simulink model "comparison_px4_mc_sim_distrb_ekf"  (R2019b)
settings: Solver=FixedStepAuto  StartTime=0.0  StopTime=sim_time  FixedStep=1/sim_freq  RelTol=1e-3
values from neighbouring files (symbols this model uses):
  C_D = [0.064; 0.067; 0.089].*0    [full_distrb_model_parameters.m]    (also in model_parameters.m)
  d = 0.11    [full_distrb_model_parameters.m]    (also in model_parameters.m)
  disturbance_rejection = 1    [full_performance_analysis.m]    (also in performance_analysis.m)
  hover_perc = m*g / max_total_T    [full_distrb_model_parameters.m]    (also in model_parameters.m)
  Ixx = 1.326e-3    (= 0.001326)    [full_distrb_model_parameters.m]    (also in model_parameters.m)
  Iyy = 9.3e-4    (= 0.00093)    [full_distrb_model_parameters.m]    (also in model_parameters.m)
  Izz = 1.95e-3    (= 0.00195)    [full_distrb_model_parameters.m]    (also in model_parameters.m)
  m = 0.66    [full_distrb_model_parameters.m]    (also in model_parameters.m)
  max_T = max_total_T / 4    [full_distrb_model_parameters.m]    (also in model_parameters.m)
  meas_noise = 0.000001    (= 1e-06)    [full_distrb_model_parameters.m]    (also in full_performance_analysis.m; model_parameters.m; noise_matrices.m = 0.0001; run_sim_full_dstrb.m)
  option1 = 3    [full_performance_analysis.m]    (also in performance_analysis.m)
  option2 = 2    [full_performance_analysis.m]    (also in performance_analysis.m = 1)
  Pk_init = zeros(15)    [full_distrb_model_parameters.m]    (also in full_performance_analysis.m; model_parameters.m = zeros(12); noise_matrices.m = zeros(12,12); run_sim_full_dstrb.m)
  pos_e_step = [0,0,0]    [full_performance_analysis.m]    (also in performance_analysis.m; run_sim.m = [0,2,0]; run_sim_full_dstrb.m)
  Qk = C22'*C12    [full_distrb_model_parameters.m]    (also in full_performance_analysis.m; model_parameters.m; noise_matrices.m; run_sim_full_dstrb.m)
  r_D = 7.997e-3    (= 0.007997)    [full_distrb_model_parameters.m]    (also in model_parameters.m)
  ramp_max = 0.15    [full_performance_analysis.m]    (also in performance_analysis.m; run_sim.m = 0.5; run_sim_full_dstrb.m = 0.1)
  ramp_slope = 0.05    [full_performance_analysis.m]    (also in performance_analysis.m; run_sim.m; run_sim_full_dstrb.m = 0.01)
  Rk = eye(9)*meas_noise    [full_distrb_model_parameters.m]    (also in full_performance_analysis.m; model_parameters.m; noise_matrices.m; run_sim_full_dstrb.m)
  sinus_amplitude = 0.2    [full_performance_analysis.m]    (also in performance_analysis.m; run_sim.m = 0.1; run_sim_full_dstrb.m = 0.1)
  sinus_bias = 0    [full_performance_analysis.m]    (also in performance_analysis.m; run_sim.m; run_sim_full_dstrb.m)
  sinus_freq = 3    [full_performance_analysis.m]    (also in performance_analysis.m = 5; run_sim.m = 1; run_sim_full_dstrb.m = 10)
  step_delay = 3    [full_performance_analysis.m]    (also in performance_analysis.m; run_sim.m = 1; run_sim_full_dstrb.m = 1)
  step_mag = 0.1    [full_performance_analysis.m]    (also in performance_analysis.m; run_sim.m = 0.5; run_sim_full_dstrb.m)
  tau_T = 0.002    [full_distrb_model_parameters.m]    (also in model_parameters.m)
  virtual_controls_mat = [1 1 1 1; -1/sqrt(2) 1/sqrt(2) 1/sqrt(2) -1/sqrt(2); 1/sqrt(2) -1/sqrt(2) 1/sqrt(2) -1/sqrt(2); 1 1 -1 -1]    [full_distrb_model_parameters.m]    (also in model_parameters.m)
  wind = [0; 0; 0]    [full_distrb_model_parameters.m]    (also in model_parameters.m)
  X_hat_init = zeros(15,1)    [full_distrb_model_parameters.m]    (also in full_performance_analysis.m; model_parameters.m = zeros(12,1); noise_matrices.m = zeros(12,1); run_sim_full_dstrb.m)
  yaw_step = 0    [full_performance_analysis.m]    (also in performance_analysis.m; run_sim.m; run_sim_full_dstrb.m)
undefined symbols (not defined in the file or in its folder): br_filt_denom, br_filt_num, DiscIntNeverNeededParam, eta_w, g, MC_PITCH_P, MC_PITCHRATE_D, MC_PITCHRATE_I, MC_PITCHRATE_MAX, MC_PITCHRATE_P, MC_PR_INT_LIM, MC_ROLL_P, MC_ROLLRATE_D, MC_ROLLRATE_I, MC_ROLLRATE_MAX, MC_ROLLRATE_P, MC_RR_INT_LIM, MC_YAW_P, MC_YAWRATE_D, MC_YAWRATE_I, MC_YAWRATE_MAX, MC_YAWRATE_P, MC_YR_INT_LIM, MPC_THR_MAX, MPC_THR_MIN, MPC_TILTMAX_AIR, MPC_XY_P, MPC_XY_VEL_D, MPC_XY_VEL_I, MPC_XY_VEL_MAX, MPC_XY_VEL_P, MPC_Z_P, MPC_Z_VEL_D, MPC_Z_VEL_I, MPC_Z_VEL_MAX_DN, MPC_Z_VEL_MAX_UP, MPC_Z_VEL_P, rho, sim_freq, vel_filt_denom, vel_filt_num
libraries: simulink x7, sharedtransform x3, shared6dof x1
settings Model: Creator=henry  LastModifiedBy=henry

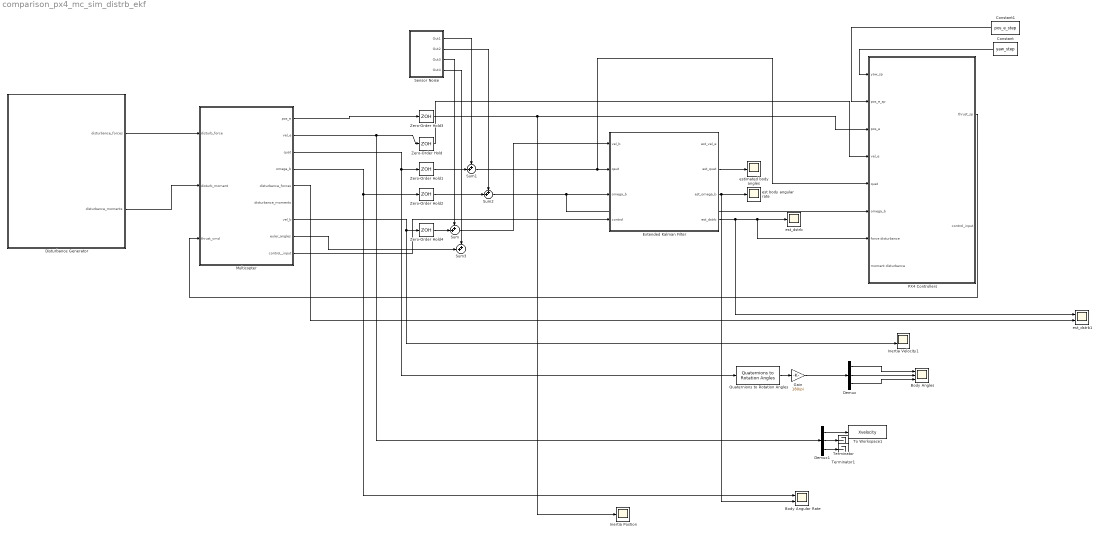
== system comparison_px4_mc_sim_distrb_ekf ==
  Body Angles : Scope  NumInputPorts=3
  Body Angular Rate : Scope  NumInputPorts=2
  Constant : Constant  Value=yaw_step
  Constant1 : Constant  Value=pos_e_step
  Demux : Demux  Outputs=3
  Demux1 : Demux  Outputs=3
  Disturbance Generator : Subsystem
  Extended Kalman Filter : Subsystem
  Gain : Gain  Gain=180/pi
  Inertia Postion : Scope
  Inertia Velocity1 : Scope  NumInputPorts=2
  Multicopter : Subsystem
  PX4 Controllers : Subsystem
  Quaternions to Rotation Angles : sharedtransform/Quaternions to Rotation Angles  rotationOrder=XYZ  aMode=aMode
      settings: SourceProductBaseCode=AE
  "Sensor Noise " : Subsystem
  Sum{,1..3} (4 alike) : Sum  Inputs=++|
  Terminator : Terminator
  Terminator1 : Terminator
  To Workspace1 : ToWorkspace  VariableName=Xvelocity  SaveFormat=Timeseries  SampleTime=-1
  Zero-Order Hold{,1..4} (5 alike) : ZeroOrderHold  SampleTime=1/sim_freq
  est body angular rate : Scope
  est_dstrb : Scope
  est_dstrb1 : Scope  NumInputPorts=2
  estimated body angles : Scope
  wires:
  Multicopter/4(omega_b) -> Body Angular Rate/1, Zero-Order Hold2/1
  Multicopter/1(pos_e) -> Zero-Order Hold3/1
  PX4 Controllers/1(thrust_sp) -> Multicopter/3(thrust_cmd)
  Constant/1 -> PX4 Controllers/1(yaw_sp)
  Constant1/1 -> PX4 Controllers/2(pos_e_sp)
  Quaternions to Rotation Angles/1 -> Gain/1
  Gain/1 -> Demux/1
  Demux/1 -> Body Angles/1
  Demux/2 -> Body Angles/2
  Demux/3 -> Body Angles/3
  Zero-Order Hold2/1 -> Sum2/2
  Sum2/1 -> PX4 Controllers/6(omega_b), Extended Kalman Filter/3(omega_b)
  Zero-Order Hold3/1 -> Inertia Postion/1, PX4 Controllers/3(pos_e)
  Multicopter/3("quat ") -> Quaternions to Rotation Angles/1, Zero-Order Hold1/1
  Multicopter/7("vel_b ") -> Inertia Velocity1/2, Zero-Order Hold4/1
  Zero-Order Hold4/1 -> Sum/2
  Sum/1 -> Extended Kalman Filter/1(vel_b)
  Zero-Order Hold/1 -> PX4 Controllers/4(vel_e)
  Extended Kalman Filter/3(est_omega_b) -> est body angular rate/1, Body Angular Rate/2
  Extended Kalman Filter/2(est_quat) -> estimated body angles/1
  Multicopter/8(euler_angles) -> Sum3/2
  Multicopter/9(controL_input) -> Extended Kalman Filter/4(control)
  Multicopter/2(vel_e) -> Demux1/1, Zero-Order Hold/1
  Zero-Order Hold1/1 -> Sum1/2
  Sum1/1 -> PX4 Controllers/5(quat), Extended Kalman Filter/2(qaut)
  Extended Kalman Filter/4(est_dstrb) -> est_dstrb1/1, PX4 Controllers/7(force disturbance), est_dstrb/1
  Multicopter/5(disturbance_forces) -> est_dstrb1/2
  Disturbance Generator/1(disturbance_forces) -> Multicopter/1(disturb_force)
  Disturbance Generator/2(disturbance_moments) -> Multicopter/2(disturb_moment)
  Demux1/2 -> Terminator/1
  Demux1/3 -> Terminator1/1
  Demux1/1 -> To Workspace1/1
  "Sensor Noise "/1(Out1) -> Sum1/1
  "Sensor Noise "/2(Out2) -> Sum2/1
  "Sensor Noise "/3(Out3) -> Sum/1
  "Sensor Noise "/4(Out4) -> Sum3/1

== system comparison_px4_mc_sim_distrb_ekf/Disturbance Generator ==
  note: RAMP
  note: DISTURBANCE TYPE
  note: STEP
  note: SINUS
  note: ACTIVATE DISTURBANCE
  MATLAB Function : MATLAB Function  TreatAsAtomicUnit=on
  Option1 : Constant  Value=option1  OutDataTypeStr=Inherit: Inherit via back propagation
  Option2 : Constant  Value=option2  OutDataTypeStr=Inherit: Inherit via back propagation
  Product : Product
  Ramp : simulink/Sources/Ramp  slope=ramp_slope  start=step_delay  InitialOutput=0
  Saturation : Saturate  UpperLimit=ramp_max  LowerLimit=0
  Sine Wave1 : Sin  Amplitude=sinus_amplitude  Bias=sinus_bias  Frequency=sinus_freq  SampleTime=0
  Step1 : Step  Time=step_delay  After=step_mag  SampleTime=0
  Step2 : Step  Time=step_delay  SampleTime=0
  activate disturbance : Constant  OutDataTypeStr=Inherit: Inherit via back propagation
  disturbance_forces : Outport
  disturbance_moments : Outport  Port=2
  wires:
  Sine Wave1/1 -> Product/1
  Step1/1 -> MATLAB Function/2(step)
  MATLAB Function/2(moments) -> disturbance_moments/1
  Product/1 -> MATLAB Function/4(sinus)
  activate disturbance/1 -> MATLAB Function/1(x)
  Option1/1 -> MATLAB Function/5(option1)
  Option2/1 -> MATLAB Function/6(option2)
  Ramp/1 -> Saturation/1
  MATLAB Function/1(forces) -> disturbance_forces/1
  Saturation/1 -> MATLAB Function/3(ramp)
  Step2/1 -> Product/2

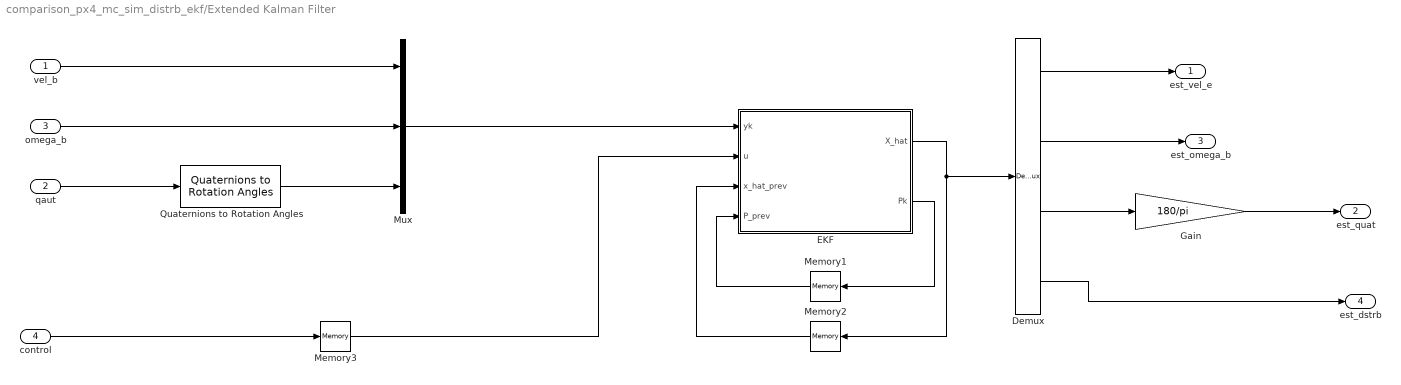
== system comparison_px4_mc_sim_distrb_ekf/Extended Kalman Filter ==
  vel_b : Inport
  qaut : Inport  Port=2
  omega_b : Inport  Port=3
  control : Inport  Port=4
  Demux : Demux
  EKF : MATLAB Function  TreatAsAtomicUnit=on
  Gain : Gain  Gain=180/pi
  Memory1 : Memory  InitialCondition=Pk_init
  Memory2 : Memory  InitialCondition=X_hat_init
  Memory3 : Memory  InitialCondition=[0 0 0 0]'
  Mux : Mux  Inputs=3
  Quaternions to Rotation Angles : sharedtransform/Quaternions to Rotation Angles  rotationOrder=XYZ  aMode=aMode
      settings: SourceProductBaseCode=AE
  est_vel_e : Outport
  est_quat : Outport  Port=2
  est_omega_b : Outport  Port=3
  est_dstrb : Outport  Port=4
  wires:
  qaut/1 -> Quaternions to Rotation Angles/1
  vel_b/1 -> Mux/1
  omega_b/1 -> Mux/2
  Mux/1 -> EKF/1(yk)
  control/1 -> Memory3/1
  Memory1/1 -> EKF/4(P_prev)
  EKF/2(Pk) -> Memory1/1
  EKF/1(X_hat) -> Memory2/1, Demux/1
  Memory2/1 -> EKF/3(x_hat_prev)
  Demux/1 -> est_vel_e/1
  Demux/2 -> est_omega_b/1
  Memory3/1 -> EKF/2(u)
  Quaternions to Rotation Angles/1 -> Mux/3
  Demux/3 -> Gain/1
  Gain/1 -> est_quat/1
  Demux/4 -> est_dstrb/1

== system comparison_px4_mc_sim_distrb_ekf/Multicopter ==
  disturb_force : Inport
  disturb_moment : Inport  Port=2
  thrust_cmd : Inport  Port=3
  6 DOF MODEL : Subsystem
  Forces and Moments : Subsystem
  Motor Model : Subsystem
  pos_e : Outport
  vel_e : Outport  Port=2
  "quat " : Outport  Port=3
  omega_b : Outport  Port=4
  disturbance_forces : Outport  Port=5
  disturbance_moments : Outport  Port=6
  "vel_b " : Outport  Port=7
  euler_angles : Outport  Port=8
  controL_input : Outport  Port=9
  wires:
  6 DOF MODEL/1(vel_b) -> "vel_b "/1, Forces and Moments/1(vel_b)
  6 DOF MODEL/3(qaut) -> Forces and Moments/3(quat), "quat "/1
  6 DOF MODEL/2(pos_e) -> pos_e/1, Forces and Moments/2(pos_e)
  Forces and Moments/2(moments) -> 6 DOF MODEL/2(moments)
  6 DOF MODEL/5(omega_b) -> omega_b/1
  6 DOF MODEL/4(vel_e) -> vel_e/1
  Forces and Moments/1(forces) -> 6 DOF MODEL/1("forces ")
  thrust_cmd/1 -> Motor Model/1(thrust_cmd)
  Motor Model/1(force) -> Forces and Moments/4(thrust_cmd)
  Forces and Moments/3(disturbance_force) -> disturbance_forces/1
  Forces and Moments/4(disturbance_moments) -> disturbance_moments/1
  disturb_force/1 -> Forces and Moments/5(disturb_force)
  disturb_moment/1 -> Forces and Moments/6(disturb_moments)
  6 DOF MODEL/6(euler_angles) -> euler_angles/1
  Forces and Moments/5(control_input) -> controL_input/1

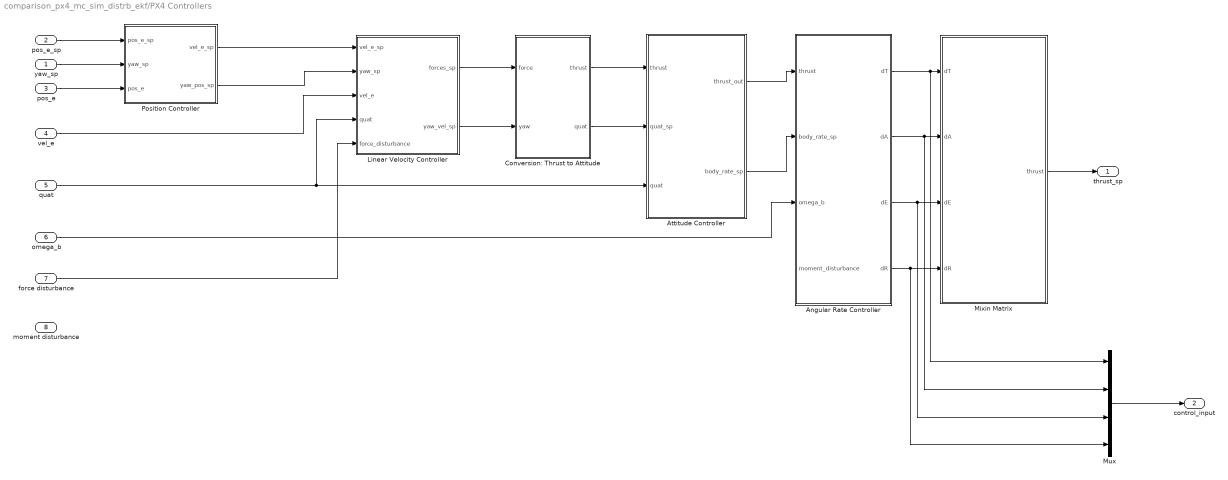
== system comparison_px4_mc_sim_distrb_ekf/PX4 Controllers ==
  yaw_sp : Inport
  pos_e_sp : Inport  Port=2
  pos_e : Inport  Port=3
  vel_e : Inport  Port=4
  quat : Inport  Port=5
  omega_b : Inport  Port=6
  force disturbance : Inport  Port=7
  moment disturbance : Inport  Port=8
  Angular Rate Controller : Subsystem
  Attitude Controller : Subsystem
  Conversion: Thrust to Attitude : Subsystem
  Linear Velocity Controller : Subsystem
  Mixin Matrix : Subsystem
  Mux : Mux
  Position Controller : Subsystem
  thrust_sp : Outport
  control_input : Outport  Port=2  PortDimensions=[4 1]
  wires:
  yaw_sp/1 -> Position Controller/2(yaw_sp)
  pos_e_sp/1 -> Position Controller/1(pos_e_sp)
  quat/1 -> Attitude Controller/3(quat), Linear Velocity Controller/4("quat ")
  omega_b/1 -> Angular Rate Controller/3(omega_b)
  pos_e/1 -> Position Controller/3(pos_e)
  vel_e/1 -> Linear Velocity Controller/3(vel_e)
  Position Controller/2(yaw_pos_sp) -> Linear Velocity Controller/2(yaw_sp)
  Position Controller/1(vel_e_sp) -> Linear Velocity Controller/1(vel_e_sp)
  Linear Velocity Controller/1(forces_sp) -> Conversion: Thrust to Attitude/1(force)
  Linear Velocity Controller/2(yaw_vel_sp) -> Conversion: Thrust to Attitude/2(yaw)
  Conversion: Thrust to Attitude/1(thrust) -> Attitude Controller/1(thrust)
  Conversion: Thrust to Attitude/2(quat) -> Attitude Controller/2(quat_sp)
  Attitude Controller/1(thrust_out) -> Angular Rate Controller/1(thrust)
  Attitude Controller/2(body_rate_sp) -> Angular Rate Controller/2(body_rate_sp)
  Angular Rate Controller/1(dT) -> Mux/1, Mixin Matrix/1(dT)
  Angular Rate Controller/2(dA) -> Mux/2, Mixin Matrix/2(dA)
  Angular Rate Controller/3(dE) -> Mux/3, Mixin Matrix/3(dE)
  Angular Rate Controller/4(dR) -> Mux/4, Mixin Matrix/4(dR)
  Mixin Matrix/1(thrust) -> thrust_sp/1
  Mux/1 -> control_input/1
  force disturbance/1 -> Linear Velocity Controller/5(force_disturbance)

== system comparison_px4_mc_sim_distrb_ekf/Sensor Noise  ==
  Random Number : RandomNumber  Mean=[ 0 0 0 ]  Variance=[meas_noise meas_noise meas_noise]  Seed=[4 5 6 ]  SampleTime=1/sim_freq  VectorParams1D=off
  Random Number1 : RandomNumber  Mean=[0 0 0]  Variance=[meas_noise meas_noise meas_noise]  Seed=[1 2 3]  SampleTime=1/sim_freq  VectorParams1D=off
  Random Number2 : RandomNumber  Mean=[0 0 0]  Variance=[meas_noise meas_noise meas_noise]  Seed=[8 9 10]  SampleTime=1/sim_freq
  Random Number3 : RandomNumber  Mean=[0 0 0 0]  Variance=[meas_noise meas_noise meas_noise meas_noise]  Seed=[11 12 13 14]  SampleTime=1/sim_freq
  Out1 : Outport
  Out2 : Outport  Port=2
  Out3 : Outport  Port=3
  Out4 : Outport  Port=4
  wires:
  Random Number3/1 -> Out1/1
  Random Number/1 -> Out4/1
  Random Number2/1 -> Out3/1
  Random Number1/1 -> Out2/1

== system comparison_px4_mc_sim_distrb_ekf/Multicopter/6 DOF MODEL ==
  "forces " : Inport
  moments : Inport  Port=2
  6DOF (Quaternion) : shared6dof/6DOF (Euler Angles)  units=Metric (MKS)  mtype=Fixed  rep=Quaternion  xme_0=[0 0 0]  Vm_0=[0 0 0]  eul_0=[0 0 0]  pm_0=[0 0 0]  mass_0=m  mass_e=0.5  mass_f=2.0  inertia=I  inertia_e=eye(3)  inertia_f=2*eye(3)  k_quat=2  vre_flag=on  abi_flag=off  aMode=0  xme_statename=''  Vm_statename=''  eul_statename=''  quat_statename=''  pm_statename=''  mass_statename=''
      settings: SourceProductBaseCode=AE
  Direction Cosine Matrix to Quaternions : sharedtransform/Direction Cosine Matrix  to Quaternions  aMode=0  action=None  tolerance=eps(2)
      settings: SourceProductName=Aerospace Blockset  SourceProductBaseCode=AE
  Terminator : Terminator
  Terminator1 : Terminator
  vel_b : Outport
  pos_e : Outport  Port=2
  qaut : Outport  Port=3
  vel_e : Outport  Port=4
  omega_b : Outport  Port=5
  euler_angles : Outport  Port=6
  wires:
  "forces "/1 -> 6DOF (Quaternion)/1
  moments/1 -> 6DOF (Quaternion)/2
  6DOF (Quaternion)/8 -> Terminator/1
  6DOF (Quaternion)/7 -> Terminator1/1
  6DOF (Quaternion)/3 -> euler_angles/1
  6DOF (Quaternion)/1 -> vel_e/1
  6DOF (Quaternion)/2 -> pos_e/1
  6DOF (Quaternion)/5 -> vel_b/1
  6DOF (Quaternion)/6 -> omega_b/1
  Direction Cosine Matrix to Quaternions/1 -> qaut/1
  6DOF (Quaternion)/4 -> Direction Cosine Matrix to Quaternions/1

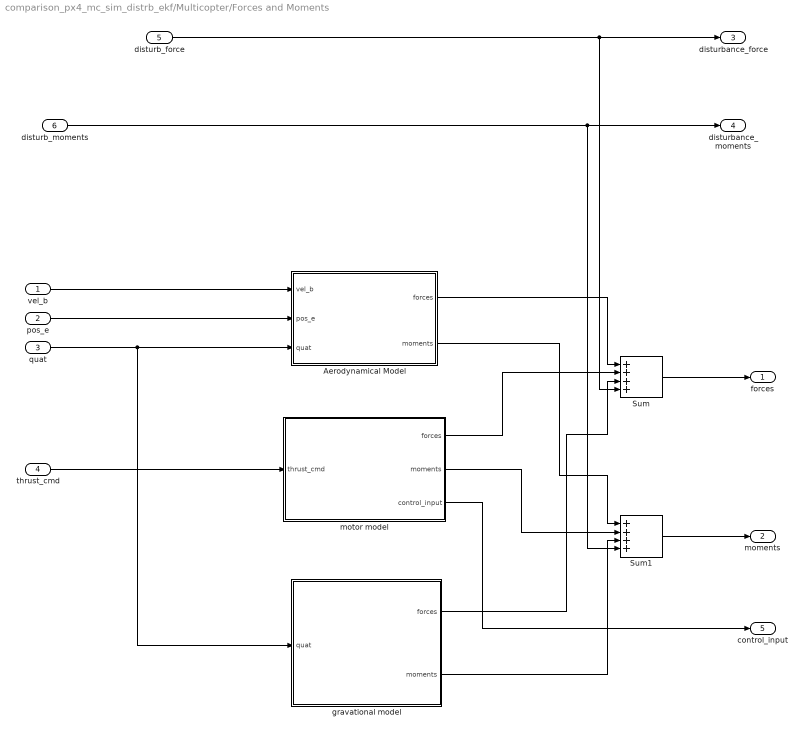
== system comparison_px4_mc_sim_distrb_ekf/Multicopter/Forces and Moments ==
  vel_b : Inport
  pos_e : Inport  Port=2
  quat : Inport  Port=3
  thrust_cmd : Inport  Port=4
  disturb_force : Inport  Port=5
  disturb_moments : Inport  Port=6
  Aerodynamical Model : Subsystem
  Sum : Sum  Inputs=++++
  Sum1 : Sum  Inputs=++++
  gravational model : Subsystem
  motor model : Subsystem
  forces : Outport
  moments : Outport  Port=2
  disturbance_force : Outport  Port=3
  disturbance_moments : Outport  Port=4
  control_input : Outport  Port=5
  wires:
  Sum/1 -> forces/1
  Sum1/1 -> moments/1
  motor model/1(forces) -> Sum/2
  motor model/2(moments) -> Sum1/2
  gravational model/1(forces) -> Sum/3
  gravational model/2(moments) -> Sum1/3
  vel_b/1 -> Aerodynamical Model/1(vel_b)
  pos_e/1 -> Aerodynamical Model/2(pos_e)
  Aerodynamical Model/1(forces) -> Sum/1
  Aerodynamical Model/2(moments) -> Sum1/1
  thrust_cmd/1 -> motor model/1(thrust_cmd)
  disturb_moments/1 -> Sum1/4, disturbance_moments/1
  quat/1 -> Aerodynamical Model/3(quat), gravational model/1(quat)
  disturb_force/1 -> Sum/4, disturbance_force/1
  motor model/3(control_input) -> control_input/1

== system comparison_px4_mc_sim_distrb_ekf/Multicopter/Motor Model ==
  thrust_cmd : Inport
  Linear Gain : Gain  Gain=max_T
  force : Outport  VectorParamsAs1DForOutWhenUnconnected=off
  wires:
  thrust_cmd/1 -> Linear Gain/1
  Linear Gain/1 -> force/1

== system comparison_px4_mc_sim_distrb_ekf/PX4 Controllers/Angular Rate Controller ==
  thrust : Inport
  body_rate_sp : Inport  Port=2
  omega_b : Inport  Port=3
  moment_disturbance : Inport  Port=4
  Demux : Demux  Outputs=3
  Demux1 : Demux  Outputs=3
  Demux2 : Demux  Outputs=3
  Pitch Rate Controller : Subsystem
  Roll Rate Controller : Subsystem
  Yaw Rate Controller : Subsystem
  dT : Outport  VectorParamsAs1DForOutWhenUnconnected=off
  dA : Outport  Port=2  VectorParamsAs1DForOutWhenUnconnected=off
  dE : Outport  Port=3  VectorParamsAs1DForOutWhenUnconnected=off
  dR : Outport  Port=4  VectorParamsAs1DForOutWhenUnconnected=off
  wires:
  Demux1/3 -> Yaw Rate Controller/2(r)
  Demux/3 -> Yaw Rate Controller/1(rref)
  Demux1/1 -> Roll Rate Controller/2(p)
  thrust/1 -> dT/1
  Yaw Rate Controller/1(dR) -> dR/1
  Pitch Rate Controller/1(dE) -> dE/1
  Demux1/2 -> Pitch Rate Controller/2(q)
  Roll Rate Controller/1(dA) -> dA/1
  Demux/1 -> Roll Rate Controller/1(pref)
  Demux/2 -> Pitch Rate Controller/1(qref)
  omega_b/1 -> Demux1/1
  body_rate_sp/1 -> Demux/1
  moment_disturbance/1 -> Demux2/1
  Demux2/2 -> Pitch Rate Controller/3(disturbance_q)
  Demux2/3 -> Yaw Rate Controller/3(disturbance_r)
  Demux2/1 -> Roll Rate Controller/3(disturbance_q)

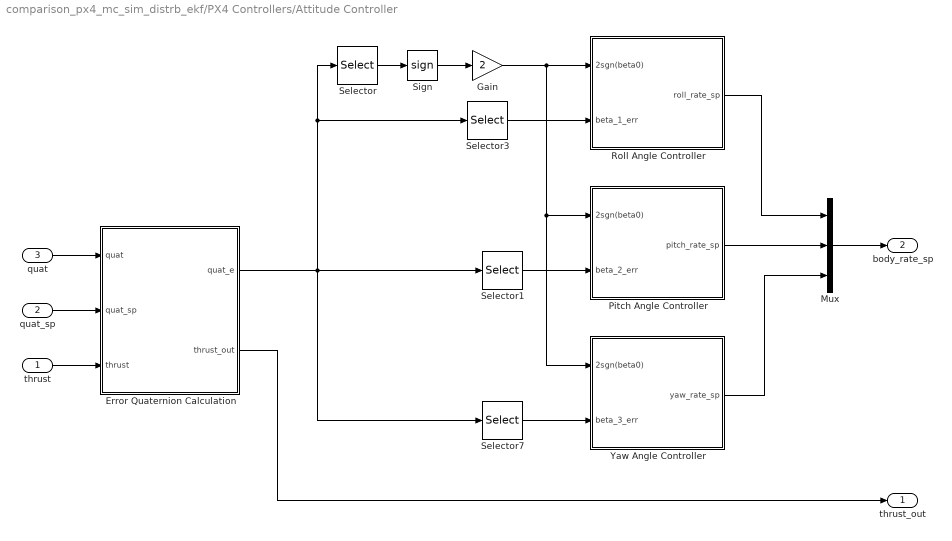
== system comparison_px4_mc_sim_distrb_ekf/PX4 Controllers/Attitude Controller ==
  thrust : Inport  PortDimensions=1
  quat_sp : Inport  Port=2  PortDimensions=4
  quat : Inport  Port=3  PortDimensions=4
  Error Quaternion Calculation : MATLAB Function  TreatAsAtomicUnit=on
  Gain : Gain  Gain=2
  Mux : Mux  Inputs=3
  Pitch Angle Controller : Subsystem
  Roll Angle Controller : Subsystem
  Selector : Selector  InputPortWidth=4  IndexOptions=Index vector (dialog)  Indices=1  OutputSizes=1
  Selector1 : Selector  InputPortWidth=4  IndexOptions=Index vector (dialog)  Indices=3  OutputSizes=1
  Selector3 : Selector  InputPortWidth=4  IndexOptions=Index vector (dialog)  Indices=2  OutputSizes=1
  Selector7 : Selector  InputPortWidth=4  IndexOptions=Index vector (dialog)  Indices=4  OutputSizes=1
  Sign : Signum
  Yaw Angle Controller : Subsystem
  thrust_out : Outport  VectorParamsAs1DForOutWhenUnconnected=off
  body_rate_sp : Outport  Port=2  VectorParamsAs1DForOutWhenUnconnected=off
  wires:
  Pitch Angle Controller/1(pitch_rate_sp) -> Mux/2
  Selector7/1 -> Yaw Angle Controller/2(beta_3_err)
  Mux/1 -> body_rate_sp/1
  quat/1 -> Error Quaternion Calculation/1(quat)
  quat_sp/1 -> Error Quaternion Calculation/2(quat_sp)
  Error Quaternion Calculation/1(quat_e) -> Selector7/1, Selector/1, Selector3/1, Selector1/1
  Selector/1 -> Sign/1
  Yaw Angle Controller/1(yaw_rate_sp) -> Mux/3
  Roll Angle Controller/1(roll_rate_sp) -> Mux/1
  Selector3/1 -> Roll Angle Controller/2(beta_1_err)
  Gain/1 -> Yaw Angle Controller/1(2sgn(beta0)), Pitch Angle Controller/1(2sgn(beta0)), Roll Angle Controller/1(2sgn(beta0))
  thrust/1 -> Error Quaternion Calculation/3(thrust)
  Sign/1 -> Gain/1
  Error Quaternion Calculation/2(thrust_out) -> thrust_out/1
  Selector1/1 -> Pitch Angle Controller/2(beta_2_err)

== system comparison_px4_mc_sim_distrb_ekf/PX4 Controllers/Conversion: Thrust to Attitude ==
  force : Inport
  yaw : Inport  Port=2
  thrust2att : MATLAB Function  TreatAsAtomicUnit=on
  thrust : Outport  VectorParamsAs1DForOutWhenUnconnected=off
  quat : Outport  Port=2  VectorParamsAs1DForOutWhenUnconnected=off
  wires:
  yaw/1 -> thrust2att/2(yaw)
  force/1 -> thrust2att/1(force)
  thrust2att/2(thrust) -> thrust/1
  thrust2att/1(quat) -> quat/1

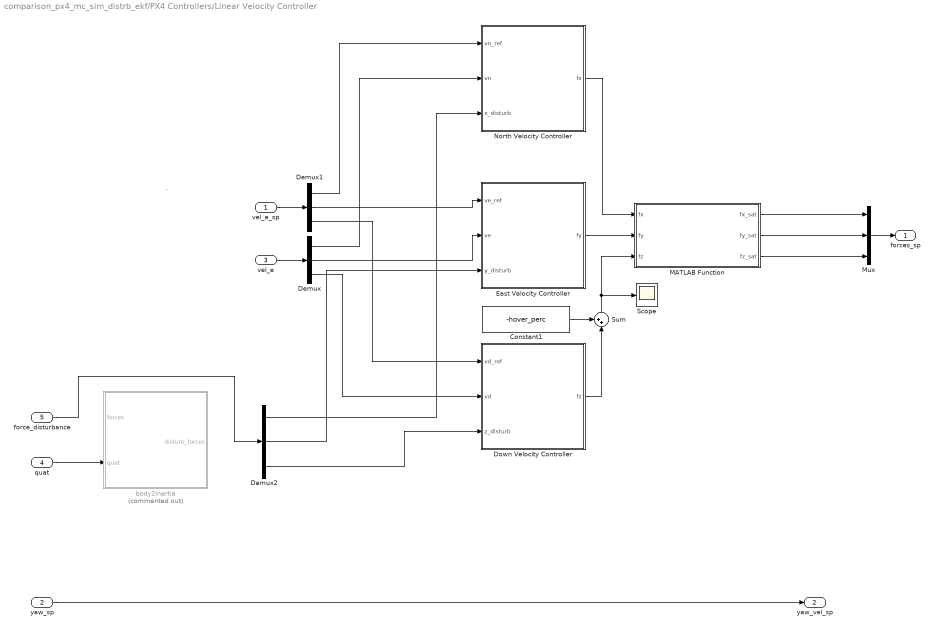
== system comparison_px4_mc_sim_distrb_ekf/PX4 Controllers/Linear Velocity Controller ==
  note: `
  vel_e_sp : Inport
  yaw_sp : Inport  Port=2
  vel_e : Inport  Port=3
  "quat " : Inport  Port=4
  force_disturbance : Inport  Port=5
  Constant1 : Constant  Value=-hover_perc
  Demux : Demux  Outputs=3
  Demux1 : Demux  Outputs=3
  Demux2 : Demux  Outputs=3
  Down Velocity Controller : Subsystem
  East Velocity Controller : Subsystem
  MATLAB Function : MATLAB Function  TreatAsAtomicUnit=on
  Mux : Mux  Inputs=3
  North Velocity Controller : Subsystem
  Scope : Scope
  Sum : Sum  Inputs=++|
  body2inertia : MATLAB Function  Commented=on  TreatAsAtomicUnit=on
  forces_sp : Outport  VectorParamsAs1DForOutWhenUnconnected=off
  yaw_vel_sp : Outport  Port=2  VectorParamsAs1DForOutWhenUnconnected=off
  wires:
  Mux/1 -> forces_sp/1
  Demux/2 -> East Velocity Controller/2(ve)
  vel_e_sp/1 -> Demux1/1
  Down Velocity Controller/1(fz) -> Sum/2
  Demux1/1 -> North Velocity Controller/1(vn_ref)
  Constant1/1 -> Sum/1
  Demux/1 -> North Velocity Controller/2(vn)
  Demux/3 -> Down Velocity Controller/2(vd)
  vel_e/1 -> Demux/1
  East Velocity Controller/1(fy) -> MATLAB Function/2(fy)
  North Velocity Controller/1(fx) -> MATLAB Function/1(fx)
  yaw_sp/1 -> yaw_vel_sp/1
  Demux1/3 -> Down Velocity Controller/1(vd_ref)
  Demux1/2 -> East Velocity Controller/1(ve_ref)
  MATLAB Function/3(fz_sat) -> Mux/3
  Sum/1 -> Scope/1, MATLAB Function/3(fz)
  MATLAB Function/2(fy_sat) -> Mux/2
  MATLAB Function/1(fx_sat) -> Mux/1
  "quat "/1 -> body2inertia/2(quat)
  Demux2/1 -> North Velocity Controller/3(x_disturb)
  force_disturbance/1 -> Demux2/1
  Demux2/2 -> East Velocity Controller/3(y_disturb)
  Demux2/3 -> Down Velocity Controller/3(z_disturb)

== system comparison_px4_mc_sim_distrb_ekf/PX4 Controllers/Mixin Matrix ==
  dT : Inport
  dA : Inport  Port=2
  dE : Inport  Port=3
  dR : Inport  Port=4
  Mixin_mat : MATLAB Function  TreatAsAtomicUnit=on
  Precision Conversion : Subsystem
  Saturation : Saturate  UpperLimit=1  LowerLimit=0
  thrust : Outport  VectorParamsAs1DForOutWhenUnconnected=off
  wires:
  Mixin_mat/1(thrust) -> Saturation/1
  dT/1 -> Mixin_mat/1(dT)
  Saturation/1 -> Precision Conversion/1(analog_cmd)
  dE/1 -> Mixin_mat/3(dE)
  dA/1 -> Mixin_mat/2(dA)
  dR/1 -> Mixin_mat/4(dR)
  Precision Conversion/1(discrete_cmd) -> thrust/1

== system comparison_px4_mc_sim_distrb_ekf/PX4 Controllers/Position Controller ==
  pos_e_sp : Inport
  yaw_sp : Inport  Port=2
  pos_e : Inport  Port=3
  Demux : Demux  Outputs=3
  Demux1 : Demux  Outputs=3
  Down Position Controller : Subsystem
  East Position Controller : Subsystem
  Mux : Mux  Inputs=3
  North Position Controller : Subsystem
  vel_e_sp : Outport  VectorParamsAs1DForOutWhenUnconnected=off
  yaw_pos_sp : Outport  Port=2  VectorParamsAs1DForOutWhenUnconnected=off
  wires:
  Demux/1 -> North Position Controller/1(n_ref)
  North Position Controller/1(vn) -> Mux/1
  pos_e_sp/1 -> Demux/1
  yaw_sp/1 -> yaw_pos_sp/1
  Demux1/1 -> North Position Controller/2(n)
  Demux/2 -> East Position Controller/1(e_ref)
  Down Position Controller/1(vd) -> Mux/3
  Demux1/2 -> East Position Controller/2(e)
  Demux/3 -> Down Position Controller/1(d_ref)
  Mux/1 -> vel_e_sp/1
  East Position Controller/1(ve) -> Mux/2
  Demux1/3 -> Down Position Controller/2(d)
  pos_e/1 -> Demux1/1

== system comparison_px4_mc_sim_distrb_ekf/Multicopter/Forces and Moments/Aerodynamical Model ==
  vel_b : Inport
  pos_e : Inport  Port=2
  quat : Inport  Port=3
  Constant : Constant  Value=wind
  aerodynamic_model : MATLAB Function  TreatAsAtomicUnit=on
  forces : Outport
  moments : Outport  Port=2
  wires:
  quat/1 -> aerodynamic_model/4(quat)
  aerodynamic_model/2(moments) -> moments/1
  vel_b/1 -> aerodynamic_model/1(v_b)
  aerodynamic_model/1(forces) -> forces/1
  pos_e/1 -> aerodynamic_model/3(ned)
  Constant/1 -> aerodynamic_model/2(vw_i)

== system comparison_px4_mc_sim_distrb_ekf/Multicopter/Forces and Moments/gravational model ==
  quat : Inport
  gravitional_model : MATLAB Function  TreatAsAtomicUnit=on
  forces : Outport
  moments : Outport  Port=2
  wires:
  gravitional_model/1(forces) -> forces/1
  gravitional_model/2(moments) -> moments/1
  quat/1 -> gravitional_model/1(quat)

== system comparison_px4_mc_sim_distrb_ekf/Multicopter/Forces and Moments/motor model ==
  thrust_cmd : Inport
  Integrator : Integrator
  Mux : Mux
  thrust_model : MATLAB Function  TreatAsAtomicUnit=on
  forces : Outport
  moments : Outport  Port=2
  control_input : Outport  Port=3
  wires:
  thrust_model/3(moments) -> moments/1
  thrust_cmd/1 -> thrust_model/2(T_cmd)
  Integrator/1 -> thrust_model/1(T)
  thrust_model/2(forces) -> forces/1
  thrust_model/1(T_dot) -> Integrator/1
  thrust_model/4(del_t) -> Mux/1
  thrust_model/5(del_a) -> Mux/2
  thrust_model/6(del_e) -> Mux/3
  thrust_model/7(del_r) -> Mux/4
  Mux/1 -> control_input/1

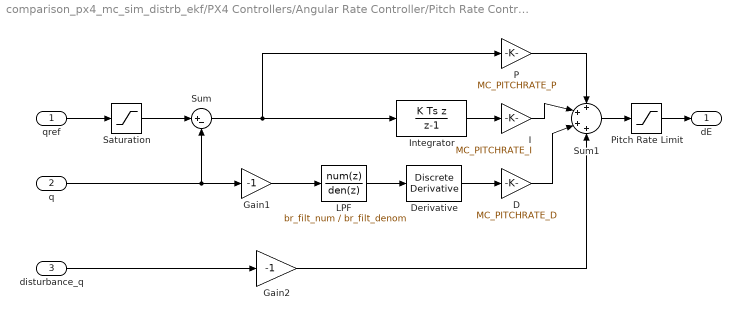
== system comparison_px4_mc_sim_distrb_ekf/PX4 Controllers/Angular Rate Controller/Pitch Rate Controller ==
  qref : Inport
  q : Inport  Port=2
  disturbance_q : Inport  Port=3
  D : Gain  Gain=MC_PITCHRATE_D
  Derivative : simulink/Discrete/Discrete Derivative  gainval=1  ICPrevScaledInput=0.0  OutMin=[]  OutMax=[]  OutDataType=fixdt(1, 16)  OutScaling=2^-10  DoSatur=off
  Gain1 : Gain  Gain=-1
  Gain2 : Gain  Gain=-1
  I : Gain  Gain=MC_PITCHRATE_I
  Integrator : DiscreteIntegrator  IntegratorMethod=Integration: Backward Euler  gainval=1  SampleTime=-1  LimitOutput=on  UpperSaturationLimit=MC_PR_INT_LIM  LowerSaturationLimit=-MC_PR_INT_LIM  ICPrevOutput=DiscIntNeverNeededParam  ICPrevScaledInput=DiscIntNeverNeededParam
  LPF : DiscreteTransferFcn  Numerator=br_filt_num  Denominator=br_filt_denom
  P : Gain  Gain=MC_PITCHRATE_P
  Pitch Rate Limit : Saturate  UpperLimit=1  LowerLimit=-1
  Saturation : Saturate  UpperLimit=MC_PITCHRATE_MAX*pi/180  LowerLimit=-MC_PITCHRATE_MAX*pi/180
  Sum : Sum  Inputs=|+-
  Sum1 : Sum  Inputs=++++
  dE : Outport  VectorParamsAs1DForOutWhenUnconnected=off
  wires:
  Gain1/1 -> LPF/1
  P/1 -> Sum1/1
  Sum1/1 -> Pitch Rate Limit/1
  Saturation/1 -> Sum/1
  I/1 -> Sum1/2
  Sum/1 -> Integrator/1, P/1
  Derivative/1 -> D/1
  D/1 -> Sum1/3
  qref/1 -> Saturation/1
  q/1 -> Gain1/1, Sum/2
  LPF/1 -> Derivative/1
  Integrator/1 -> I/1
  Pitch Rate Limit/1 -> dE/1
  disturbance_q/1 -> Gain2/1
  Gain2/1 -> Sum1/4

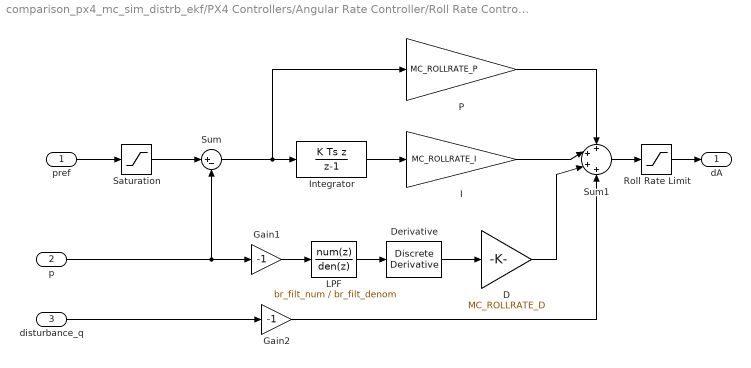
== system comparison_px4_mc_sim_distrb_ekf/PX4 Controllers/Angular Rate Controller/Roll Rate Controller ==
  pref : Inport
  p : Inport  Port=2
  disturbance_q : Inport  Port=3
  D : Gain  Gain=MC_ROLLRATE_D
  Derivative : simulink/Discrete/Discrete Derivative  gainval=1  ICPrevScaledInput=0.0  OutMin=[]  OutMax=[]  OutDataType=fixdt(1, 16)  OutScaling=2^-10  DoSatur=off
  Gain1 : Gain  Gain=-1
  Gain2 : Gain  Gain=-1
  I : Gain  Gain=MC_ROLLRATE_I
  Integrator : DiscreteIntegrator  IntegratorMethod=Integration: Backward Euler  gainval=1  SampleTime=-1  LimitOutput=on  UpperSaturationLimit=MC_RR_INT_LIM  LowerSaturationLimit=-MC_RR_INT_LIM  ICPrevOutput=DiscIntNeverNeededParam  ICPrevScaledInput=DiscIntNeverNeededParam
  LPF : DiscreteTransferFcn  Numerator=br_filt_num  Denominator=br_filt_denom
  P : Gain  Gain=MC_ROLLRATE_P
  Roll Rate Limit : Saturate  UpperLimit=1  LowerLimit=-1
  Saturation : Saturate  UpperLimit=MC_ROLLRATE_MAX*pi/180  LowerLimit=-MC_ROLLRATE_MAX*pi/180
  Sum : Sum  Inputs=|+-
  Sum1 : Sum  Inputs=++++
  dA : Outport  VectorParamsAs1DForOutWhenUnconnected=off
  wires:
  Gain1/1 -> LPF/1
  P/1 -> Sum1/1
  Sum1/1 -> Roll Rate Limit/1
  Saturation/1 -> Sum/1
  I/1 -> Sum1/2
  Sum/1 -> P/1, Integrator/1
  Derivative/1 -> D/1
  D/1 -> Sum1/3
  pref/1 -> Saturation/1
  p/1 -> Gain1/1, Sum/2
  LPF/1 -> Derivative/1
  Integrator/1 -> I/1
  Roll Rate Limit/1 -> dA/1
  disturbance_q/1 -> Gain2/1
  Gain2/1 -> Sum1/4

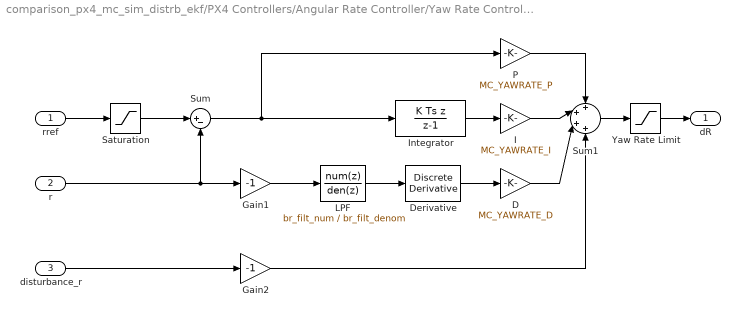
== system comparison_px4_mc_sim_distrb_ekf/PX4 Controllers/Angular Rate Controller/Yaw Rate Controller ==
  rref : Inport
  r : Inport  Port=2
  disturbance_r : Inport  Port=3
  D : Gain  Gain=MC_YAWRATE_D
  Derivative : simulink/Discrete/Discrete Derivative  gainval=1  ICPrevScaledInput=0.0  OutMin=[]  OutMax=[]  OutDataType=fixdt(1, 16)  OutScaling=2^-10  DoSatur=off
  Gain1 : Gain  Gain=-1
  Gain2 : Gain  Gain=-1
  I : Gain  Gain=MC_YAWRATE_I
  Integrator : DiscreteIntegrator  IntegratorMethod=Integration: Backward Euler  gainval=1  SampleTime=-1  LimitOutput=on  UpperSaturationLimit=MC_YR_INT_LIM  LowerSaturationLimit=-MC_YR_INT_LIM  ICPrevOutput=DiscIntNeverNeededParam  ICPrevScaledInput=DiscIntNeverNeededParam
  LPF : DiscreteTransferFcn  Numerator=br_filt_num  Denominator=br_filt_denom
  P : Gain  Gain=MC_YAWRATE_P
  Saturation : Saturate  UpperLimit=MC_YAWRATE_MAX*pi/180  LowerLimit=-MC_YAWRATE_MAX*pi/180
  Sum : Sum  Inputs=|+-
  Sum1 : Sum  Inputs=++++
  Yaw Rate Limit : Saturate  UpperLimit=1  LowerLimit=-1
  dR : Outport  VectorParamsAs1DForOutWhenUnconnected=off
  wires:
  Gain1/1 -> LPF/1
  P/1 -> Sum1/1
  Sum1/1 -> Yaw Rate Limit/1
  Saturation/1 -> Sum/1
  I/1 -> Sum1/2
  Sum/1 -> Integrator/1, P/1
  Derivative/1 -> D/1
  D/1 -> Sum1/3
  rref/1 -> Saturation/1
  r/1 -> Gain1/1, Sum/2
  LPF/1 -> Derivative/1
  Integrator/1 -> I/1
  Yaw Rate Limit/1 -> dR/1
  disturbance_r/1 -> Gain2/1
  Gain2/1 -> Sum1/4

== system comparison_px4_mc_sim_distrb_ekf/PX4 Controllers/Attitude Controller/Pitch Angle Controller ==
  2sgn(beta0) : Inport
  beta_2_err : Inport  Port=2
  Multiply : Product
  P : Gain  Gain=MC_PITCH_P
  pitch_rate_sp : Outport  VectorParamsAs1DForOutWhenUnconnected=off
  wires:
  P/1 -> Multiply/1
  beta_2_err/1 -> P/1
  2sgn(beta0)/1 -> Multiply/2
  Multiply/1 -> pitch_rate_sp/1

== system comparison_px4_mc_sim_distrb_ekf/PX4 Controllers/Attitude Controller/Roll Angle Controller ==
  2sgn(beta0) : Inport
  beta_1_err : Inport  Port=2
  Multiply : Product
  P : Gain  Gain=MC_ROLL_P
  roll_rate_sp : Outport  VectorParamsAs1DForOutWhenUnconnected=off
  wires:
  P/1 -> Multiply/1
  beta_1_err/1 -> P/1
  2sgn(beta0)/1 -> Multiply/2
  Multiply/1 -> roll_rate_sp/1

== system comparison_px4_mc_sim_distrb_ekf/PX4 Controllers/Attitude Controller/Yaw Angle Controller ==
  2sgn(beta0) : Inport
  beta_3_err : Inport  Port=2
  Multiply : Product
  P : Gain  Gain=MC_YAW_P
  yaw_rate_sp : Outport  VectorParamsAs1DForOutWhenUnconnected=off
  wires:
  P/1 -> Multiply/1
  beta_3_err/1 -> P/1
  2sgn(beta0)/1 -> Multiply/2
  Multiply/1 -> yaw_rate_sp/1

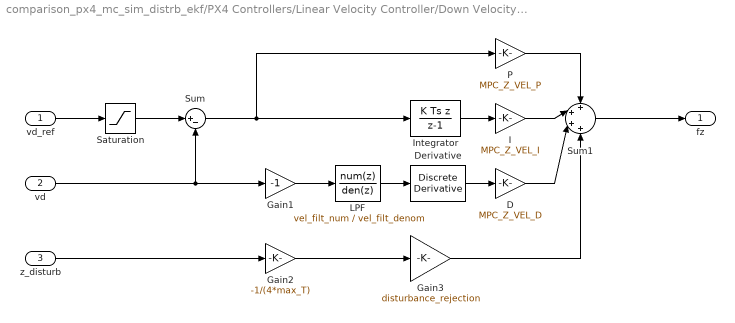
== system comparison_px4_mc_sim_distrb_ekf/PX4 Controllers/Linear Velocity Controller/Down Velocity Controller ==
  vd_ref : Inport
  vd : Inport  Port=2
  z_disturb : Inport  Port=3
  D : Gain  Gain=MPC_Z_VEL_D
  Derivative : simulink/Discrete/Discrete Derivative  gainval=1  ICPrevScaledInput=0.0  OutMin=[]  OutMax=[]  OutDataType=fixdt(1, 16)  OutScaling=2^-10  DoSatur=off
  Gain1 : Gain  Gain=-1
  Gain2 : Gain  Gain=-1/(4*max_T)
  Gain3 : Gain  Gain=disturbance_rejection
  I : Gain  Gain=MPC_Z_VEL_I
  Integrator : DiscreteIntegrator  IntegratorMethod=Integration: Backward Euler  gainval=1  SampleTime=-1  UpperSaturationLimit=MC_PR_INT_LIM  LowerSaturationLimit=-MC_PR_INT_LIM  ICPrevOutput=DiscIntNeverNeededParam  ICPrevScaledInput=DiscIntNeverNeededParam
  LPF : DiscreteTransferFcn  Numerator=vel_filt_num  Denominator=vel_filt_denom
  P : Gain  Gain=MPC_Z_VEL_P
  Saturation : Saturate  UpperLimit=MPC_Z_VEL_MAX_UP  LowerLimit=-MPC_Z_VEL_MAX_DN
  Sum : Sum  Inputs=|+-
  Sum1 : Sum  Inputs=++++
  fz : Outport  VectorParamsAs1DForOutWhenUnconnected=off
  wires:
  vd_ref/1 -> Saturation/1
  P/1 -> Sum1/1
  Sum1/1 -> fz/1
  vd/1 -> Sum/2, Gain1/1
  Gain1/1 -> LPF/1
  LPF/1 -> Derivative/1
  D/1 -> Sum1/3
  Saturation/1 -> Sum/1
  I/1 -> Sum1/2
  Integrator/1 -> I/1
  Sum/1 -> Integrator/1, P/1
  Derivative/1 -> D/1
  z_disturb/1 -> Gain2/1
  Gain2/1 -> Gain3/1
  Gain3/1 -> Sum1/4

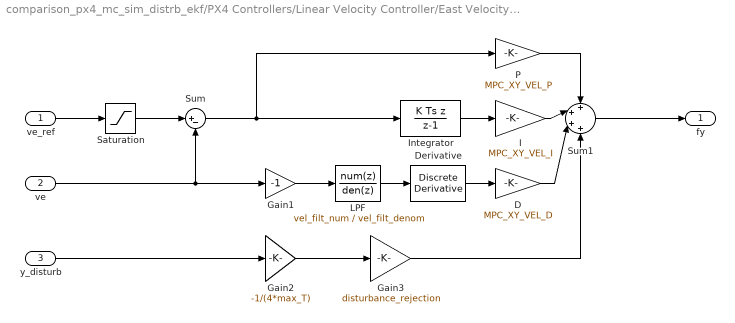
== system comparison_px4_mc_sim_distrb_ekf/PX4 Controllers/Linear Velocity Controller/East Velocity Controller ==
  ve_ref : Inport
  ve : Inport  Port=2
  y_disturb : Inport  Port=3
  D : Gain  Gain=MPC_XY_VEL_D
  Derivative : simulink/Discrete/Discrete Derivative  gainval=1  ICPrevScaledInput=0.0  OutMin=[]  OutMax=[]  OutDataType=fixdt(1, 16)  OutScaling=2^-10  DoSatur=off
  Gain1 : Gain  Gain=-1
  Gain2 : Gain  Gain=-1/(4*max_T)
  Gain3 : Gain  Gain=disturbance_rejection
  I : Gain  Gain=MPC_XY_VEL_I
  Integrator : DiscreteIntegrator  IntegratorMethod=Integration: Backward Euler  gainval=1  SampleTime=-1  UpperSaturationLimit=MC_PR_INT_LIM  LowerSaturationLimit=-MC_PR_INT_LIM  ICPrevOutput=DiscIntNeverNeededParam  ICPrevScaledInput=DiscIntNeverNeededParam
  LPF : DiscreteTransferFcn  Numerator=vel_filt_num  Denominator=vel_filt_denom
  P : Gain  Gain=MPC_XY_VEL_P
  Saturation : Saturate  UpperLimit=MPC_XY_VEL_MAX  LowerLimit=-MPC_XY_VEL_MAX
  Sum : Sum  Inputs=|+-
  Sum1 : Sum  Inputs=++++
  fy : Outport  VectorParamsAs1DForOutWhenUnconnected=off
  wires:
  ve_ref/1 -> Saturation/1
  P/1 -> Sum1/1
  Sum1/1 -> fy/1
  ve/1 -> Sum/2, Gain1/1
  Gain1/1 -> LPF/1
  LPF/1 -> Derivative/1
  D/1 -> Sum1/3
  Saturation/1 -> Sum/1
  I/1 -> Sum1/2
  Integrator/1 -> I/1
  Sum/1 -> Integrator/1, P/1
  Derivative/1 -> D/1
  y_disturb/1 -> Gain2/1
  Gain2/1 -> Gain3/1
  Gain3/1 -> Sum1/4

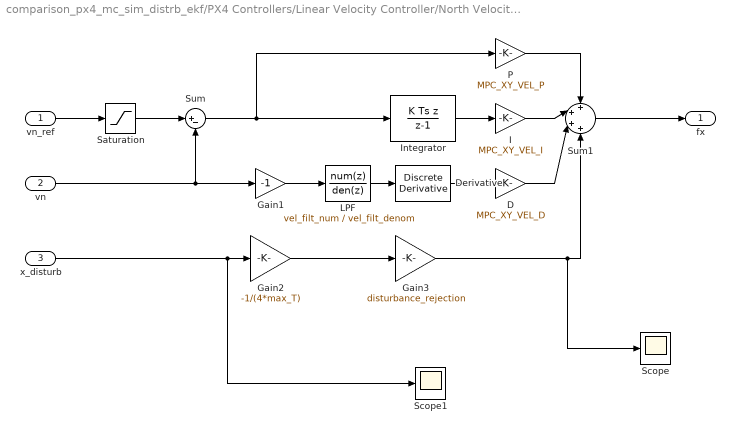
== system comparison_px4_mc_sim_distrb_ekf/PX4 Controllers/Linear Velocity Controller/North Velocity Controller ==
  vn_ref : Inport
  vn : Inport  Port=2
  x_disturb : Inport  Port=3
  D : Gain  Gain=MPC_XY_VEL_D
  Derivative : simulink/Discrete/Discrete Derivative  gainval=1  ICPrevScaledInput=0.0  OutMin=[]  OutMax=[]  OutDataType=fixdt(1, 16)  OutScaling=2^-10  DoSatur=off
  Gain1 : Gain  Gain=-1
  Gain2 : Gain  Gain=-1/(4*max_T)
  Gain3 : Gain  Gain=disturbance_rejection
  I : Gain  Gain=MPC_XY_VEL_I
  Integrator : DiscreteIntegrator  IntegratorMethod=Integration: Backward Euler  gainval=1  SampleTime=-1  UpperSaturationLimit=MC_PR_INT_LIM  LowerSaturationLimit=-MC_PR_INT_LIM  ICPrevOutput=DiscIntNeverNeededParam  ICPrevScaledInput=DiscIntNeverNeededParam
  LPF : DiscreteTransferFcn  Numerator=vel_filt_num  Denominator=vel_filt_denom
  P : Gain  Gain=MPC_XY_VEL_P
  Saturation : Saturate  UpperLimit=MPC_XY_VEL_MAX  LowerLimit=-MPC_XY_VEL_MAX
  Scope : Scope
  Scope1 : Scope
  Sum : Sum  Inputs=|+-
  Sum1 : Sum  Inputs=++++
  fx : Outport  VectorParamsAs1DForOutWhenUnconnected=off
  wires:
  vn_ref/1 -> Saturation/1
  P/1 -> Sum1/1
  Sum1/1 -> fx/1
  vn/1 -> Sum/2, Gain1/1
  LPF/1 -> Derivative/1
  D/1 -> Sum1/3
  Saturation/1 -> Sum/1
  I/1 -> Sum1/2
  Integrator/1 -> I/1
  Sum/1 -> Integrator/1, P/1
  Derivative/1 -> D/1
  Gain1/1 -> LPF/1
  Gain2/1 -> Gain3/1
  Gain3/1 -> Scope/1, Sum1/4
  x_disturb/1 -> Scope1/1, Gain2/1

== system comparison_px4_mc_sim_distrb_ekf/PX4 Controllers/Mixin Matrix/Precision Conversion ==
  analog_cmd : Inport
  Gain : Gain  Gain=10000
  Gain1 : Gain  Gain=1/10000
  Round : Rounding
  discrete_cmd : Outport  VectorParamsAs1DForOutWhenUnconnected=off
  wires:
  analog_cmd/1 -> Gain/1
  Gain/1 -> Round/1
  Round/1 -> Gain1/1
  Gain1/1 -> discrete_cmd/1

== system comparison_px4_mc_sim_distrb_ekf/PX4 Controllers/Position Controller/Down Position Controller ==
  d_ref : Inport
  d : Inport  Port=2
  P : Gain  Gain=MPC_Z_P
  Sum : Sum  Inputs=|+-
  vd : Outport  VectorParamsAs1DForOutWhenUnconnected=off
  wires:
  d/1 -> Sum/2
  d_ref/1 -> Sum/1
  Sum/1 -> P/1
  P/1 -> vd/1

== system comparison_px4_mc_sim_distrb_ekf/PX4 Controllers/Position Controller/East Position Controller ==
  e_ref : Inport
  e : Inport  Port=2
  P : Gain  Gain=MPC_XY_P
  Sum : Sum  Inputs=|+-
  ve : Outport  VectorParamsAs1DForOutWhenUnconnected=off
  wires:
  e/1 -> Sum/2
  e_ref/1 -> Sum/1
  Sum/1 -> P/1
  P/1 -> ve/1

== system comparison_px4_mc_sim_distrb_ekf/PX4 Controllers/Position Controller/North Position Controller ==
  n_ref : Inport
  n : Inport  Port=2
  P : Gain  Gain=MPC_XY_P
  Sum : Sum  Inputs=|+-
  vn : Outport  VectorParamsAs1DForOutWhenUnconnected=off
  wires:
  n/1 -> Sum/2
  n_ref/1 -> Sum/1
  Sum/1 -> P/1
  P/1 -> vn/1

== matlab function comparison_px4_mc_sim_distrb_ekf/Multicopter/Forces and Moments/motor model/thrust_model ==
  data: T input; T_cmd input; T_dot output; forces output; moments output; virtual_controls_mat parameter; tau_T parameter; d parameter; r_D parameter; del_t output; del_a output; del_e output; del_r output
function [T_dot, forces, moments,del_t,del_a,del_e,del_r] = thrust_model(T, T_cmd,virtual_controls_mat,tau_T, d,r_D)

    virt_T = virtual_controls_mat * T;

    T_dot = (-T + T_cmd)/tau_T;
    forces = [0; 0; -virt_T(1)];
    moments = [d*virt_T(2); d*virt_T(3); r_D*virt_T(4)];
    del_t = virt_T(1);
    del_a = virt_T(2);
    del_e = virt_T(3);
    del_r = virt_T(4);
    
end

== matlab function comparison_px4_mc_sim_distrb_ekf/Multicopter/Forces and Moments/Aerodynamical Model/aerodynamic_model ==
  data: v_b input; forces output; vw_i input; ned input; quat input; moments output; rho parameter; C_D parameter; eta_w parameter
function [forces,moments] = aerodynamic_model(v_b, vw_i, ned, quat, rho, C_D, eta_w)
    coder.extrinsic("quatrotate");
    
    % Initialize
    vw_b = [0; 0; 0];
    
    vw_b = quatrotate(quat', vw_i')';
    vw_bm = (power(abs(ned(3))/10, eta_w)) .* vw_b;
    v_bw = -v_b + vw_bm;
    q = 0.5 * rho * v_bw.*abs(v_bw);
    
    forces = q.*C_D;
    moments = [0; 0; 0];
    
end

== matlab function comparison_px4_mc_sim_distrb_ekf/Multicopter/Forces and Moments/gravational model/gravitional_model ==
  data: quat input; forces output; moments output; g parameter; m parameter
function [forces,moments] = gravitional_model(quat, g, m)
    coder.extrinsic("quatrotate");

    % Initialize
    forces = [0; 0; 0];
    
    moments = [0 ; 0 ; 0];
    forces = quatrotate(quat', [0 ; 0 ; m*g]')';

end

== matlab function comparison_px4_mc_sim_distrb_ekf/PX4 Controllers/Linear Velocity Controller/MATLAB Function ==
  data: fx input; fx_sat output; fy input; fz input; fy_sat output; fz_sat output; MPC_THR_MAX parameter; MPC_THR_MIN parameter; MPC_TILTMAX_AIR parameter
function [fx_sat, fy_sat, fz_sat] = constrain_max_tilt(fx, fy, fz,MPC_THR_MAX, MPC_THR_MIN,MPC_TILTMAX_AIR)
    % First constrain fz.
    if fz > -MPC_THR_MIN
        fz_sat = -MPC_THR_MIN;
    elseif fz < -MPC_THR_MAX
        fz_sat = -MPC_THR_MAX;
    else
        fz_sat = fz;
    end
    
    % Constrain fx and fy
    thrust_max_NE_tilt = abs(fz_sat) * tan(MPC_TILTMAX_AIR * pi/180);
    thrust_max_NE = sqrt(MPC_THR_MAX*MPC_THR_MAX - fz_sat*fz_sat);
    thrust_max_NE = min(thrust_max_NE_tilt, thrust_max_NE);
    
    fx_sat = fx;
    fy_sat = fy;
    
    if dot([fx, fy], [fx, fy]) > thrust_max_NE*thrust_max_NE
        mag = norm([fx, fy]);
        fx_sat = fx / mag * thrust_max_NE;
        fy_sat = fy / mag * thrust_max_NE;
    end
end

== matlab function comparison_px4_mc_sim_distrb_ekf/PX4 Controllers/Conversion: Thrust to Attitude/thrust2att ==
  data: force input size=3; quat output size=4; yaw input size=1; thrust output size=1
function [quat, thrust] = thrust2att(force, yaw)
    coder.extrinsic('dcm2quat');

% Read: Minimum  Snap  Trajectory  Generation  and  Control  for
% Quadrotors by Daniel Mellinger and Vijay Kumar to understand

        % Initialise quat
    quat = [1; 0; 0; 0];
    
    % Thrust is norm of force
    thrust = norm(force);
    
    % Determine body_z rotation (fit body_z onto z axis of force)
    if thrust > 1e-6
        body_z = -force./thrust;
    else
       body_z = [0; 0; 1]; 
    end
    
    % Determine body_x
    yaw_dir = [-sin(yaw); cos(yaw); 0];
    
    if abs(body_z(3)) > 1e-6
        body_x = cross(yaw_dir, body_z);
        
        if body_z(3) < 0
            body_x = -body_x;
        end
        body_x = body_x ./ norm(body_x);
    else
        body_x = [0; 0; 1];
    end
    
    % Determine body_y
    body_y = cross(body_z, body_x);
    body_y = body_y ./ norm(body_y);
    
    % Calculate rotation
    dcm = [body_x body_y body_z];
    quat = dcm2quat(dcm');
    
    % Normalise quaternion
    quat = quat ./ norm(quat);
    
end

== matlab function comparison_px4_mc_sim_distrb_ekf/PX4 Controllers/Attitude Controller/Error Quaternion Calculation ==
  data: quat input; quat_sp input; quat_e output; thrust input; thrust_out output
function [quat_e, thrust_out] = error_quat(quat, quat_sp, thrust)
    if quat_sp == [0; 0; 0; 0]
       quat_sp = [1; 0; 0; 0];
    end
    
    quat_e = quatmultiply([quat(1) -quat(2) -quat(3) -quat(4)]./norm(quat), quat_sp');
    thrust_out = thrust;
end

== matlab function comparison_px4_mc_sim_distrb_ekf/PX4 Controllers/Mixin Matrix/Mixin_mat ==
  data: dT input; thrust output; dA input; dE input; dR input; mixin_matrix parameter
function thrust = mixin_mat(dT, dA, dE, dR, mixin_matrix)

    thrust = mixin_matrix * [dT; dA; dE; dR];

end

== matlab function comparison_px4_mc_sim_distrb_ekf/PX4 Controllers/Linear Velocity Controller/body2inertia ==
  data: forces input; disturb_forces output; quat input
function disturb_forces  = body2Inertia(forces,quat)
    coder.extrinsic("quatrotate");
    coder.extrinsic("quatinv");

    disturb_forces = [0;0;0];
    
    disturb_forces = quatrotate(quatinv(quat'), forces');
    
end

== matlab function comparison_px4_mc_sim_distrb_ekf/Disturbance Generator/MATLAB Function ==
  data: x input; forces output; moments output; step input; ramp input; sinus input; option1 input; option2 input
function [forces,moments] = fcn(x,step,ramp,sinus,option1,option2)
    % x : activate disturbance
    % y : activate disturbance rejection
    % z : disturbance type selector
    % a : disturbance moment selector
    % b : disturbance force selector
    % options1: disturbance type
        % 1 step, 2 ramp, 3 sinus
    % options2: force or moment
        % 1 force, 2 moment
        
        
    forces= [0;0;0];
    moments = [0;0;0];
%     option1
%     option2
    if x
        % Moments
        if option2 == 1
            forces = [1;0;0];
        elseif option2 == 2
            moments = [0;1;0];
        end
        
    else
        forces= [0;0;0];
        moments = [0;0;0];
    end
    
    if option1 == 1
        forces = step*forces;
        moments = step*moments;
    elseif option1 == 2
        forces = ramp*forces;
        moments = ramp*moments;
    elseif option1 == 3
        forces = sinus*forces;
        moments = sinus*moments;          
    end
%     forces
%     moments

    
end

== matlab function comparison_px4_mc_sim_distrb_ekf/Extended Kalman Filter/EKF ==
  data: yk input size=[1 9]; u input size=[4 1]; X_hat output size=[12 1]; x_hat_prev input size=[12, 1]; P_prev input size=[12 12]; Pk output size=[12 12]; Qk parameter size=[12 12]; Rk parameter size=[9 9]; m parameter; g parameter; Ixx parameter; Iyy parameter; Izz parameter; r_D parameter; d parameter
function [X_hat,Pk]= fcn(yk,u,x_hat_prev,P_prev,Qk, Rk,m, g, Ixx, Iyy, Izz, r_D, d)

U=x_hat_prev(1);
V=x_hat_prev(2);
W=x_hat_prev(3);
P=x_hat_prev(4);
Q=x_hat_prev(5);
R=x_hat_prev(6);
phi=x_hat_prev(7);
theta=x_hat_prev(8);
psi=x_hat_prev(9);
Fx=x_hat_prev(10);
Fy=x_hat_prev(11);
Fz=x_hat_prev(12);

del_t=u(1);
del_a=u(2);
del_e=u(3);
del_r=u(4);

yk=yk';

F = @(U,V,W,P,Q,R,phi,theta,psi,del_t,del_a,del_e,del_r,Fx,Fy,Fz)[
[                            R*V - Q*W + (Fx - g*m*sin(theta))/m]
[                   P*W - R*U + (Fy + g*m*cos(theta)*sin(phi))/m]
[ Q*U - P*V + (Fz - del_t - d*del_a + g*m*cos(phi)*cos(theta))/m]
[                          (d*del_a)/Ixx + (Q*R*(Iyy - Izz))/Ixx]
[                          (d*del_e)/Iyy - (P*R*(Ixx - Izz))/Iyy]
[                        (del_r*r_D)/Izz + (P*Q*(Ixx - Izz))/Izz]
[              P + R*cos(phi)*tan(theta) + Q*sin(phi)*tan(theta)]
[                                        Q*cos(phi) - R*sin(phi)]
[              (R*cos(phi))/cos(theta) + (Q*sin(phi))/cos(theta)]
[                                                              0]
[                                                              0]
[                                                              0]
];
           
           
 %% Jacobian
 Fk = @(U,V,W,P,Q,R,phi,theta,psi,Fx,Fy,Fz) [
[      1,  R/250, -Q/250,                          0,                    -W/250,                      V/250,                                                             0,                                                                     -(g*cos(theta))/250, 0, 1/(250*m),         0,         0]
[ -R/250,      1,  P/250,                      W/250,                         0,                     -U/250,                                   (g*cos(phi)*cos(theta))/250,                                                            -(g*sin(phi)*sin(theta))/250, 0,         0, 1/(250*m),         0]
[  Q/250, -P/250,      1,                     -V/250,                     U/250,                          0,                                  -(g*cos(theta)*sin(phi))/250,                                                            -(g*cos(phi)*sin(theta))/250, 0,         0,         0, 1/(250*m)]
[      0,      0,      0,                          1, (R*(Iyy - Izz))/(250*Ixx),  (Q*(Iyy - Izz))/(250*Ixx),                                                             0,                                                                                       0, 0,         0,         0,         0]
[      0,      0,      0, -(R*(Ixx - Izz))/(250*Iyy),                         1, -(P*(Ixx - Izz))/(250*Iyy),                                                             0,                                                                                       0, 0,         0,         0,         0]
[      0,      0,      0,  (Q*(Ixx - Izz))/(250*Izz), (P*(Ixx - Izz))/(250*Izz),                          1,                                                             0,                                                                                       0, 0,         0,         0,         0]
[      0,      0,      0,                      1/250, (sin(phi)*tan(theta))/250,  (cos(phi)*tan(theta))/250, (Q*cos(phi)*tan(theta))/250 - (R*sin(phi)*tan(theta))/250 + 1,               (R*cos(phi)*(tan(theta)^2 + 1))/250 + (Q*sin(phi)*(tan(theta)^2 + 1))/250, 0,         0,         0,         0]
[      0,      0,      0,                          0,              cos(phi)/250,              -sin(phi)/250,                         - (R*cos(phi))/250 - (Q*sin(phi))/250,                                                                                       1, 0,         0,         0,         0]
[      0,      0,      0,                          0, sin(phi)/(250*cos(theta)),  cos(phi)/(250*cos(theta)), (Q*cos(phi))/(250*cos(theta)) - (R*sin(phi))/(250*cos(theta)), (R*cos(phi)*sin(theta))/(250*cos(theta)^2) + (Q*sin(phi)*sin(theta))/(250*cos(theta)^2), 1,         0,         0,         0]
[      0,      0,      0,                          0,                         0,                          0,                                                             0,                                                                                       0, 0,         1,         0,         0]
[      0,      0,      0,                          0,                         0,                          0,                                                             0,                                                                                       0, 0,         0,         1,         0]
[      0,      0,      0,                          0,                         0,                          0,                                                             0,                                                                                       0, 0,         0,         0,         1]
];
%% Control Update
Pk_ =  Fk(U,V,W,P,Q,R,phi,theta,psi,Fx,Fy,Fz) * P_prev * transpose( Fk(U,V,W,P,Q,R,phi,theta,psi,Fx,Fy,Fz) ) + Qk;
Xk_ = x_hat_prev + F(U,V,W,P,Q,R,phi,theta,psi,del_t,del_a,del_e,del_r,Fx,Fy,Fz)*1/250; 
         
Hk = eye(9,12);
%% Measurement Update
Lk = Pk_*transpose(Hk)*inv(Hk*Pk_*transpose(Hk) + Rk);
Pk = (eye(12) - Lk*Hk)*Pk_;
X_hat = Xk_ + Lk*(yk - Hk*Xk_);
